simulink library "MSP_FSW_lib"  (R2016b)
settings: Solver=VariableStepAuto  StartTime=0.0  StopTime=10.0  RelTol=1e-3
undefined symbols (not defined in the file): cmd_MT_fsw_dv, sc_mode, states, target
libraries: bus_stubs_fsw x2, CAN_out_lib x1, extended_kalman_filter_lib x1, actuator_processing x1, command_generation x1, env_estimation_lib x1, mode_selection x1, sensor_processing_fsw_lib x1, target_generation_lib x1
settings Model: Creator=taylorreynolds  LastModifiedBy=taylorreynolds

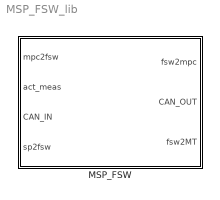
== system MSP_FSW_lib ==
  MSP_FSW : Subsystem

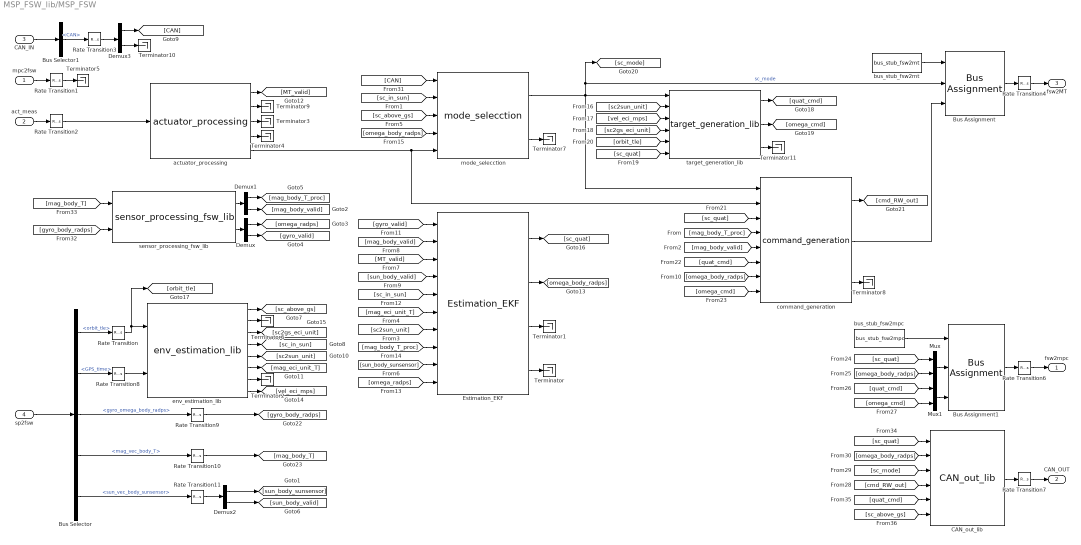
== system MSP_FSW_lib/MSP_FSW ==
  mpc2fsw : Inport  OutDataTypeStr=Bus: mpc2fsw
  act_meas : Inport  Port=2
  CAN_IN : Inport  Port=3  OutDataTypeStr=Bus: CAN_IN
  sp2fsw : Inport  Port=4  OutDataTypeStr=Bus: sp2fsw
  Bus Assignment : BusAssignment  AssignedSignals=sc_mode,cmd_MT_fsw_dv
  Bus Assignment1 : BusAssignment  AssignedSignals=states,target
  Bus Selector : BusSelector  OutputSignals=orbit_tle,GPS_time,gyro_omega_body_radps,mag_vec_body_T,sun_vec_body_sunsensor
  Bus Selector1 : BusSelector  OutputSignals=CAN
  CAN_out_lib : CAN_out_lib/CAN_out_lib
  Demux : Demux  Outputs=[3 1]
  Demux1 : Demux  Outputs=[3 1]
  Demux2 : Demux  Outputs=[3 1]
  Demux3 : Demux  Outputs=[7 1]
  "Estimation_EKF " : extended_kalman_filter_lib/Estimation_EKF 
  Mux : Mux  Inputs=[4 3]
  Mux1 : Mux  Inputs=[4 3]
  Rate Transition : RateTransition  X0=fsw_params.environment.sgp4.orbit_tle  OutPortSampleTime=fsw_params.sample_time_s
  Rate Transition{1..3,9..11} (6 alike) : RateTransition  OutPortSampleTime=fsw_params.sample_time_s
  Rate Transition4 : RateTransition
  Rate Transition6 : RateTransition
  Rate Transition7 : RateTransition
  Rate Transition8 : RateTransition  X0=fsw_params.sensor_processing.gps.ic.time  OutPortSampleTime=fsw_params.sample_time_s
  Terminator{,1..11} (12 alike) : Terminator
  actuator_processing : actuator_processing/actuator_processing
  bus_stub_fsw2mpc : bus_stubs_fsw/bus_stub_fsw2mpc
  bus_stub_fsw2mt : bus_stubs_fsw/bus_stub_fsw2mt
  command_generation : command_generation/command_generation
  env_estimation_lib : env_estimation_lib/env_estimation_lib
  mode_selecction : mode_selection/mode_selecction
  sensor_processing_fsw_lib : sensor_processing_fsw_lib/sensor_processing_fsw_lib
  target_generation_lib : target_generation_lib/target_generation_lib
  fsw2mpc : Outport
  CAN_OUT : Outport  Port=2
  fsw2MT : Outport  Port=3
  wires:
  Rate Transition3/1 -> Demux3/1
  Bus Selector1/1 -> Rate Transition3/1  "<CAN>"
  [omega_body_radps] -> command_generation/7
  Rate Transition11/1 -> Demux2/1
  Rate Transition10/1 -> [mag_body_T]
  Rate Transition9/1 -> [gyro_body_radps]
  Rate Transition8/1 -> env_estimation_lib/2
  Rate Transition/1 -> [orbit_tle], env_estimation_lib/1
  Bus Selector/1 -> Rate Transition/1  "<orbit_tle>"
  [sc_above_gs] -> mode_selecction/3
  env_estimation_lib/1 -> [sc_above_gs]
  "Estimation_EKF "/1 -> [sc_quat]
  command_generation/3 -> Terminator8/1
  command_generation/2 -> Bus Assignment/3
  command_generation/1 -> [cmd_RW_out]
  [mag_body_valid] -> command_generation/5
  [mag_body_T_proc] -> command_generation/4
  [sc2sun_unit] -> "Estimation_EKF "/7
  [mag_eci_unit_T] -> "Estimation_EKF "/6
  [mag_body_T_proc] -> "Estimation_EKF "/8
  [sun_body_sunsensor] -> "Estimation_EKF "/9
  [omega_radps] -> "Estimation_EKF "/10
  env_estimation_lib/3 -> [sc2gs_eci_unit]
  env_estimation_lib/2 -> Terminator6/1
  env_estimation_lib/8 -> [vel_eci_mps]
  actuator_processing/4 -> Terminator4/1
  actuator_processing/3 -> Terminator3/1
  env_estimation_lib/7 -> Terminator2/1
  env_estimation_lib/6 -> [mag_eci_unit_T]
  env_estimation_lib/5 -> [sc2sun_unit]
  "Estimation_EKF "/3 -> Terminator1/1
  "Estimation_EKF "/4 -> Terminator/1
  [sc_in_sun] -> "Estimation_EKF "/5
  [sun_body_valid] -> "Estimation_EKF "/4
  [MT_valid] -> "Estimation_EKF "/3
  env_estimation_lib/4 -> [sc_in_sun]
  [gyro_valid] -> "Estimation_EKF "/1
  [mag_body_valid] -> "Estimation_EKF "/2
  [sc_in_sun] -> mode_selecction/2
  mode_selecction/1 -> [sc_mode], Bus Assignment/2, command_generation/1, target_generation_lib/1  "sc_mode"
  Bus Selector/3 -> Rate Transition9/1  "<gyro_omega_body_radps>"
  Demux/1 -> [omega_radps]
  Demux/2 -> [gyro_valid]
  Bus Selector/4 -> Rate Transition10/1  "<mag_vec_body_T>"
  Demux1/1 -> [mag_body_T_proc]
  Demux1/2 -> [mag_body_valid]
  Bus Selector/5 -> Rate Transition11/1  "<sun_vec_body_sunsensor>"
  Demux2/1 -> [sun_body_sunsensor]
  Demux2/2 -> [sun_body_valid]
  act_meas/1 -> Rate Transition2/1
  actuator_processing/1 -> [MT_valid]
  actuator_processing/2 -> Terminator9/1
  Bus Selector/2 -> Rate Transition8/1  "<GPS_time>"
  "Estimation_EKF "/2 -> [omega_body_radps]
  actuator_processing/5 -> command_generation/2, mode_selecction/5
  [omega_body_radps] -> mode_selecction/4
  [sc2sun_unit] -> target_generation_lib/2
  [vel_eci_mps] -> target_generation_lib/3
  [sc2gs_eci_unit] -> target_generation_lib/4
  [sc_quat] -> target_generation_lib/6
  [orbit_tle] -> target_generation_lib/5
  [sc_quat] -> command_generation/3
  target_generation_lib/1 -> [quat_cmd]
  target_generation_lib/2 -> [omega_cmd]
  [quat_cmd] -> command_generation/6
  [omega_cmd] -> command_generation/8
  mpc2fsw/1 -> Rate Transition1/1
  mode_selecction/2 -> Terminator7/1
  bus_stub_fsw2mt/1 -> Bus Assignment/1
  Bus Assignment/1 -> Rate Transition4/1
  Bus Assignment1/1 -> Rate Transition6/1
  bus_stub_fsw2mpc/1 -> Bus Assignment1/1
  [sc_quat] -> Mux/1
  [omega_body_radps] -> Mux/2
  Mux/1 -> Bus Assignment1/2
  [quat_cmd] -> Mux1/1
  [omega_cmd] -> Mux1/2
  Mux1/1 -> Bus Assignment1/3
  CAN_out_lib/1 -> Rate Transition7/1
  sp2fsw/1 -> Bus Selector/1
  Rate Transition1/1 -> Terminator5/1
  Rate Transition2/1 -> actuator_processing/1
  CAN_IN/1 -> Bus Selector1/1
  Rate Transition4/1 -> fsw2MT/1
  Rate Transition6/1 -> fsw2mpc/1
  Rate Transition7/1 -> CAN_OUT/1
  Demux3/1 -> [CAN]
  Demux3/2 -> Terminator10/1
  [CAN] -> mode_selecction/1
  sensor_processing_fsw_lib/2 -> Demux/1
  sensor_processing_fsw_lib/1 -> Demux1/1
  [gyro_body_radps] -> sensor_processing_fsw_lib/2
  [mag_body_T] -> sensor_processing_fsw_lib/1
  [cmd_RW_out] -> CAN_out_lib/4
  [sc_mode] -> CAN_out_lib/3
  [omega_body_radps] -> CAN_out_lib/2
  [sc_quat] -> CAN_out_lib/1
  [quat_cmd] -> CAN_out_lib/5
  [sc_above_gs] -> CAN_out_lib/6
  target_generation_lib/3 -> Terminator11/1
